simulink model "EENG417_P2_EstimatorandintegratorwithNonlinearmodelsubsys"  (R2024b)
settings: Solver=VariableStepAuto  StartTime=0.0  StopTime=10.0  RelTol=1e-3
settings Model: Creator=jelly  LastModifiedBy=jelly

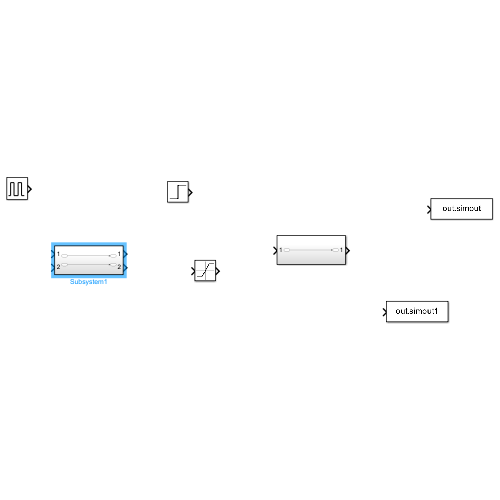
[thumbnail: Simulink's stored preview of the top-level diagram]
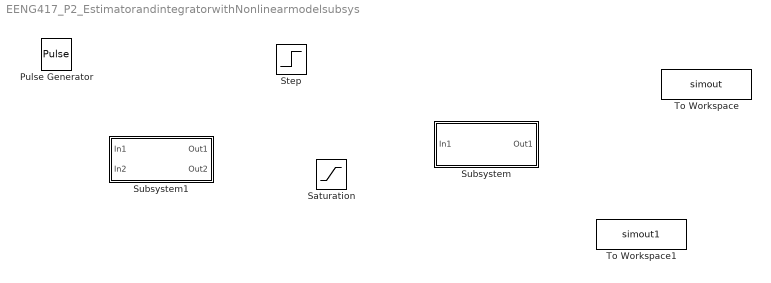
== system EENG417_P2_EstimatorandintegratorwithNonlinearmodelsubsys ==
  Pulse Generator : DiscretePulseGenerator  PulseType=Time based  Period=10  PulseWidth=5
  Saturation : Saturate
  Step : Step  SampleTime=0
  Subsystem : Subsystem
  Subsystem1 : Subsystem
  To Workspace : ToWorkspace  VariableName=simout  SaveFormat=Timeseries  SampleTime=-1
  To Workspace1 : ToWorkspace  VariableName=simout1  SaveFormat=Timeseries  SampleTime=-1

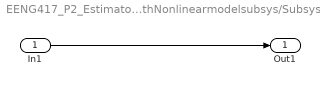
== system EENG417_P2_EstimatorandintegratorwithNonlinearmodelsubsys/Subsystem ==
  In1 : Inport
  Out1 : Outport
  wires:
  In1/1 -> Out1/1

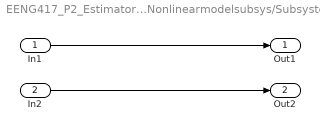
== system EENG417_P2_EstimatorandintegratorwithNonlinearmodelsubsys/Subsystem1 ==
  In1 : Inport
  In2 : Inport  Port=2
  Out1 : Outport
  Out2 : Outport  Port=2
  wires:
  In1/1 -> Out1/1
  In2/1 -> Out2/1
